simulink model "KociolPom1CvwCvgCvs"  (Simulink 7.6)
settings: Solver=ode45  SolverMode=SingleTasking  StartTime=0.0  StopTime=3000  MaxStep=1  RelTol=1e-3  AbsTol=1e-6
values from neighbouring files (symbols this model uses):
  cpw = 4190    [aparam1.m]
  Cvg = (no*Vg)*row*cpw/skala    (= 3421.83333333)    [aparam1.m]
  Cvk = (Vk)*row*cpw/skala    (= 3421.83333333)    [aparam1.m]
  Cvs = (no*Vs)*ros*cps/skala    (= 52500)    [aparam1.m]
  Cvw = (no*Vw)*rop*cpp/skala    [aparam1.m]
  czas_skok = 500    [2punktowazn.m]    (also in KociolPom1CvwCvgCvs_skrypt.m; KociolPom1CvwCvg_skrypt.m; kociolsimulinkskokjednostkowy.m; stycznazn.m)
  dFg = 0*FgN    [2punktowazn.m]    (also in KociolPom1CvwCvgCvs_skrypt.m; KociolPom1CvwCvg_skrypt.m; kociolsimulinkskokjednostkowy.m = 0; stycznazn.m)
  dQk = 0.1 * QkN    (= 200)    [2punktowazn.m]    (also in KociolPom1CvwCvgCvs_skrypt.m; KociolPom1CvwCvg_skrypt.m = 400; kociolsimulinkskokjednostkowy.m; stycznazn.m = 0)
  dQt = 0    [2punktowazn.m]    (also in KociolPom1CvwCvgCvs_skrypt.m; KociolPom1CvwCvg_skrypt.m; kociolsimulinkskokjednostkowy.m; stycznazn.m = 200)
  dTzew = 0    [2punktowazn.m]    (also in KociolPom1CvwCvgCvs_skrypt.m; KociolPom1CvwCvg_skrypt.m; kociolsimulinkskokjednostkowy.m; stycznazn.m)
  Fg0 = FgN    [2punktowazn.m]    (also in KociolPom1CvwCvgCvs_skrypt.m; KociolPom1CvwCvg_skrypt.m; kociolsimulinkskokjednostkowy.m; stycznazn.m)
  Kcg = QgN/(TgpN-TwewN)    (= 40)    [2punktowazn.m]    (also in KociolPom1CvwCvgCvs_skrypt.m; KociolPom1CvwCvg_skrypt.m; kociolsimulinkskokjednostkowy.m; stycznazn.m)
  Kcs = QgN/(TsN-TzewN)    (= 80)    [KociolPom1CvwCvgCvs_skrypt.m]
  Kcw = QgN/(TwewN-TzewN)    (= 50)    [2punktowazn.m]    (also in KociolPom1CvwCvgCvs_skrypt.m = 133.333333333; KociolPom1CvwCvg_skrypt.m; kociolsimulinkskokjednostkowy.m; stycznazn.m)
  Qk0 = QkN    (= 2000)    [2punktowazn.m]    (also in KociolPom1CvwCvgCvs_skrypt.m; KociolPom1CvwCvg_skrypt.m = 0; kociolsimulinkskokjednostkowy.m; stycznazn.m)
  Qt0 = 0    [2punktowazn.m]    (also in KociolPom1CvwCvgCvs_skrypt.m; KociolPom1CvwCvg_skrypt.m; kociolsimulinkskokjednostkowy.m; stycznazn.m)
  Tgp0 = x0(2)    [2punktowazn.m]    (also in KociolPom1CvwCvgCvs_skrypt.m; KociolPom1CvwCvg_skrypt.m; kociolsimulinkskokjednostkowy.m = 70; stycznazn.m = 70)
  Tkz0 = x0(3)    [2punktowazn.m]    (also in KociolPom1CvwCvgCvs_skrypt.m = x0(4); KociolPom1CvwCvg_skrypt.m; kociolsimulinkskokjednostkowy.m = Qk0/(cpw*Fk0) + Tgp0; stycznazn.m = Qk0/(cpw*Fk0) + Tgp0)
  To = 20*60/skala    (= 20)    [aparam1.m]
  Ts0 = x0(3)    [KociolPom1CvwCvgCvs_skrypt.m]
  Twew0 = x0(1)    [2punktowazn.m]    (also in KociolPom1CvwCvgCvs_skrypt.m; KociolPom1CvwCvg_skrypt.m; kociolsimulinkskokjednostkowy.m = 20; stycznazn.m = 20)
  Tzew0 = TzewN+0    (= -20)    [2punktowazn.m]    (also in KociolPom1CvwCvgCvs_skrypt.m; KociolPom1CvwCvg_skrypt.m; kociolsimulinkskokjednostkowy.m; stycznazn.m)
settings Model: Creator=ac  LastModifiedBy=ac  ExtModeTrigMode=oneshot  ExtModeArmWhenConnect=off
settings DataIOCC: LimitDataPoints=off
settings OptimizationCC: BlockReduction=off  BooleanDataType=off
settings DebuggingCC: SaveWithParameterizedLinksMsg=none  SignalResolutionControl=TryResolveAllWithWarning  SolverPrmCheckMsg=none  MultiTaskDSMMsg=warning  MultiTaskCondExecSysMsg=none  StrictBusMsg=None
settings HardwareCC: TargetUnknown=on
settings RTWCC: IncludeERTFirstTime=on

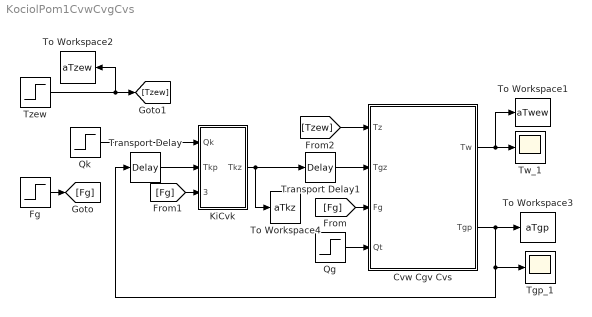
== system KociolPom1CvwCvgCvs ==
  Cvw Cgv Cvs : Subsystem
  Fg : Step  Time=czas_skok  Before=Fg0  After=Fg0+dFg  SampleTime=0
  KiCvk : Subsystem  mask{cpw=cpw, Cvk=Cvk, Tkz0=Tkz0}
  Qg : Step  Time=czas_skok  Before=Qt0  After=Qt0+dQt  SampleTime=0
  Qk : Step  Time=czas_skok  Before=Qk0  After=Qk0+dQk  SampleTime=0
  Tgp_1 : Scope
  To Workspace1 : ToWorkspace  VariableName=aTwew  SampleTime=-1  SaveFormat=Array
  To Workspace2 : ToWorkspace  VariableName=aTzew  SampleTime=-1  SaveFormat=Array
  To Workspace3 : ToWorkspace  VariableName=aTgp  SampleTime=-1  SaveFormat=Array
  To Workspace4 : ToWorkspace  VariableName=aTkz  SampleTime=-1  SaveFormat=Array
  Transport Delay : TransportDelay  DelayTime=To  InitialOutput=Tgp0
  Transport Delay1 : TransportDelay  DelayTime=To  InitialOutput=Tkz0
  Tw_1 : Scope
  Tzew : Step  Time=czas_skok  Before=Tzew0  After=Tzew0+dTzew  SampleTime=0
  wires:
  [Fg] -> KiCvk/3(Fgm)
  Transport Delay/1 -> KiCvk/2(Tkp)
  Tzew/1 -> To Workspace2/1, [Tzew]
  Qk/1 -> KiCvk/1(Qk)
  Fg/1 -> [Fg]
  Qg/1 -> Cvw Cgv Cvs/4(Qt)
  Cvw Cgv Cvs/1(Tw) -> Tw_1/1, To Workspace1/1
  Cvw Cgv Cvs/2(Tgp) -> To Workspace3/1, Tgp_1/1, Transport Delay/1
  [Fg] -> Cvw Cgv Cvs/3(Fg)
  Transport Delay1/1 -> Cvw Cgv Cvs/2(Tgz)
  [Tzew] -> Cvw Cgv Cvs/1(Tz)
  KiCvk/1(Tkz) -> Transport Delay1/1, To Workspace4/1

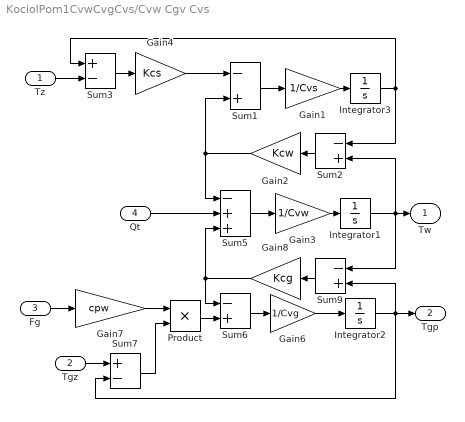
== system KociolPom1CvwCvgCvs/Cvw Cgv Cvs ==
  Tz : Inport
  Tgz : Inport  Port=2
  Fg : Inport  Port=3
  Qt : Inport  Port=4
  Gain1 : Gain  Gain=1/Cvs  SaturateOnIntegerOverflow=on  OutDataTypeStr=Inherit: Same as input  ParamDataTypeStr=Inherit: Same as input
  Gain2 : Gain  Gain=Kcw  SaturateOnIntegerOverflow=on  OutDataTypeStr=Inherit: Same as input  ParamDataTypeStr=Inherit: Same as input
  Gain3 : Gain  Gain=1/Cvw  SaturateOnIntegerOverflow=on  OutDataTypeStr=Inherit: Same as input  ParamDataTypeStr=Inherit: Same as input
  Gain4 : Gain  Gain=Kcs  SaturateOnIntegerOverflow=on  OutDataTypeStr=Inherit: Same as input  ParamDataTypeStr=Inherit: Same as input
  Gain6 : Gain  Gain=1/Cvg  SaturateOnIntegerOverflow=on  OutDataTypeStr=Inherit: Same as input  ParamDataTypeStr=Inherit: Same as input
  Gain7 : Gain  Gain=cpw  SaturateOnIntegerOverflow=on  OutDataTypeStr=Inherit: Same as input  ParamDataTypeStr=Inherit: Same as input
  Gain8 : Gain  Gain=Kcg  SaturateOnIntegerOverflow=on  OutDataTypeStr=Inherit: Same as input  ParamDataTypeStr=Inherit: Same as input
  Integrator1 : Integrator  InitialCondition=Twew0
  Integrator2 : Integrator  InitialCondition=Tgp0
  Integrator3 : Integrator  InitialCondition=Ts0
  Product : Product  SaturateOnIntegerOverflow=on  RndMeth=Zero  InputSameDT=on  OutDataTypeStr=Inherit: Same as first input
  Sum{1..2,6,9} (4 alike) : Sum  Inputs=-+  SaturateOnIntegerOverflow=on  InputSameDT=on  OutDataTypeStr=Inherit: Same as first input
  Sum3 : Sum  Inputs=+-  SaturateOnIntegerOverflow=on  InputSameDT=on  OutDataTypeStr=Inherit: Same as first input
  Sum5 : Sum  Inputs=-++  SaturateOnIntegerOverflow=on  InputSameDT=on  OutDataTypeStr=Inherit: Same as first input
  Sum7 : Sum  Inputs=+-  SaturateOnIntegerOverflow=on  InputSameDT=on  OutDataTypeStr=Inherit: Same as first input
  Tw : Outport
  Tgp : Outport  Port=2
  wires:
  Sum5/1 -> Gain3/1
  Sum6/1 -> Gain6/1
  Gain7/1 -> Product/1
  Sum7/1 -> Product/2
  Product/1 -> Sum6/2
  Gain6/1 -> Integrator2/1
  Integrator2/1 -> Sum7/2, Sum9/2, Tgp/1
  Sum9/1 -> Gain8/1
  Gain3/1 -> Integrator1/1
  Integrator1/1 -> Sum9/1, Tw/1, Sum2/2
  Gain8/1 -> Sum6/1, Sum5/3
  Fg/1 -> Gain7/1
  Tgz/1 -> Sum7/1
  Sum1/1 -> Gain1/1
  Gain1/1 -> Integrator3/1
  Sum2/1 -> Gain2/1
  Integrator3/1 -> Sum2/1, Sum3/1
  Tz/1 -> Sum3/2
  Sum3/1 -> Gain4/1
  Gain4/1 -> Sum1/1
  Gain2/1 -> Sum1/2, Sum5/1
  Qt/1 -> Sum5/2

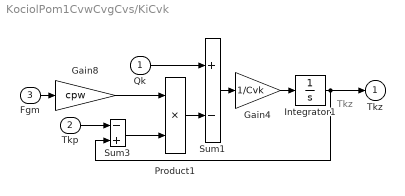
== system KociolPom1CvwCvgCvs/KiCvk ==
  note: Tkz
  Qk : Inport
  Tkp : Inport  Port=2
  Fgm : Inport  Port=3
  Gain4 : Gain  Gain=1/Cvk  SaturateOnIntegerOverflow=on  OutDataTypeStr=Inherit: Same as input  ParamDataTypeStr=Inherit: Same as input
  Gain8 : Gain  Gain=cpw  SaturateOnIntegerOverflow=on  OutDataTypeStr=Inherit: Same as input  ParamDataTypeStr=Inherit: Same as input
  Integrator1 : Integrator  InitialCondition=Tkz0
  Product1 : Product  Inputs=**  SaturateOnIntegerOverflow=on  RndMeth=Zero  InputSameDT=on  OutDataTypeStr=Inherit: Same as first input
  Sum1 : Sum  Inputs=+-  SaturateOnIntegerOverflow=on  InputSameDT=on  OutDataTypeStr=Inherit: Same as first input
  Sum3 : Sum  Inputs=-+  SaturateOnIntegerOverflow=on  InputSameDT=on  OutDataTypeStr=Inherit: Same as first input
  Tkz : Outport
  wires:
  Tkp/1 -> Sum3/1
  Integrator1/1 -> Sum3/2, Tkz/1
  Product1/1 -> Sum1/2
  Sum1/1 -> Gain4/1
  Gain4/1 -> Integrator1/1
  Qk/1 -> Sum1/1
  Gain8/1 -> Product1/1
  Sum3/1 -> Product1/2
  Fgm/1 -> Gain8/1
